simulink model "infasning"  (R2020a)
settings: Solver=VariableStepAuto  StartTime=0.0  StopTime=1  MaxStep=1e-4  RelTol=1e-3
settings Model: Creator=ielolof  LastModifiedBy=98all
settings DataIOCC: ReturnWorkspaceOutputs=off
settings DebuggingCC: ArithmeticOperatorsInVariantConditions=warning
settings SFSimCC: SimUseLocalCustomCode=off  CustomCodeUndefinedFunction=UseInterfaceOnly
settings RTWCC: RTWUseLocalCustomCode=off

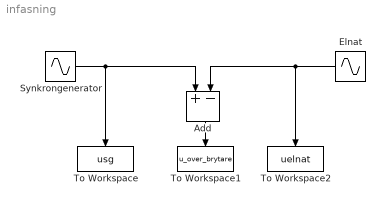
== system infasning ==
  Add : Sum  Inputs=+-
  Elnat : Sin  Amplitude=sqrt(2)*220  Frequency=2*pi*50  SampleTime=0
  Synkrongenerator : Sin  Amplitude=sqrt(2)*220*0.95  Frequency=2*pi*50*1.05  SampleTime=0
  To Workspace : ToWorkspace  VariableName=usg  SampleTime=-1
  To Workspace1 : ToWorkspace  VariableName=u_over_brytare  SampleTime=-1
  To Workspace2 : ToWorkspace  VariableName=uelnat  SampleTime=-1
  wires:
  Synkrongenerator/1 -> To Workspace/1, Add/1
  Elnat/1 -> To Workspace2/1, Add/2
  Add/1 -> To Workspace1/1
